simulink model "V4_Modell_EM_Validierung"  (R2022b)
settings: Solver=VariableStepAuto  StartTime=0.0  StopTime=10.0  RelTol=1e-3
values from neighbouring files (symbols this model uses):
  r_ZR = 0.021    [V4_Parameter_Parameter_komplett_te.m]    (also in V4_Parameter_Wagen_Te.m; V4_Parameter_komplett.m)
settings Model: Creator=JSCHB  LastModifiedBy=JSCHB

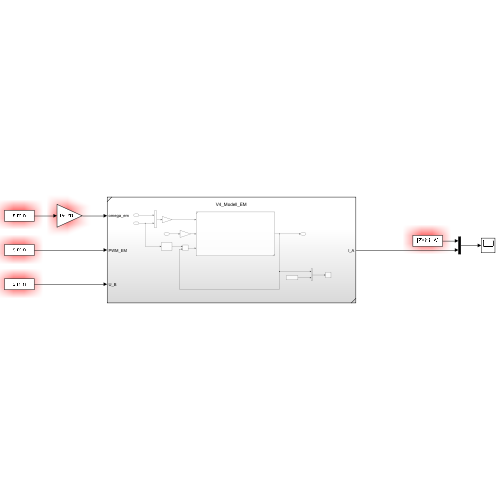
[thumbnail: Simulink's stored preview of the top-level diagram]
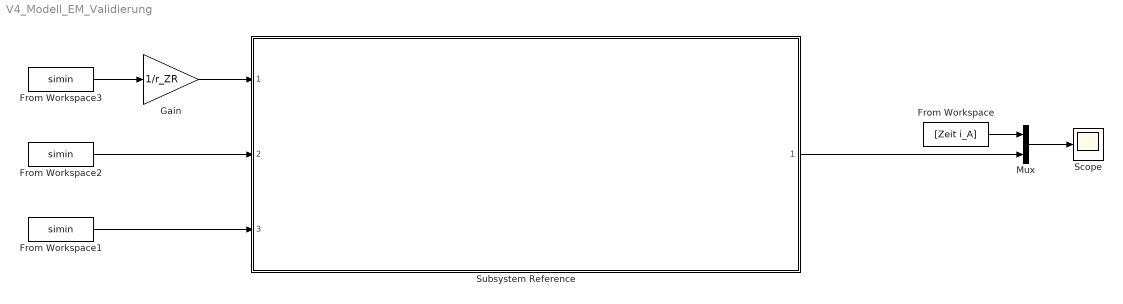
== system V4_Modell_EM_Validierung ==
  From Workspace : FromWorkspace  VariableName=[Zeit i_A]
  From Workspace1 : FromWorkspace  VariableName=simin
  From Workspace2 : FromWorkspace  VariableName=simin
  From Workspace3 : FromWorkspace  VariableName=simin
  Gain : Gain  Gain=1/r_ZR
  Mux : Mux  Inputs=2
  Scope : Scope
  Subsystem Reference : Subsystem  ReferencedSubsystem=V4_Modell_EM
  wires:
  Subsystem Reference/1 -> Mux/2
  From Workspace/1 -> Mux/1
  Mux/1 -> Scope/1
  From Workspace2/1 -> Subsystem Reference/2
  From Workspace1/1 -> Subsystem Reference/3
  From Workspace3/1 -> Gain/1
  Gain/1 -> Subsystem Reference/1
